simulink subsystem "simplePitch"  (R2024b)
settings: Solver=VariableStepAuto  StartTime=0.0  StopTime=10.0  RelTol=1e-3
settings Model: Creator=flyingtopher  LastModifiedBy=flyingtopher

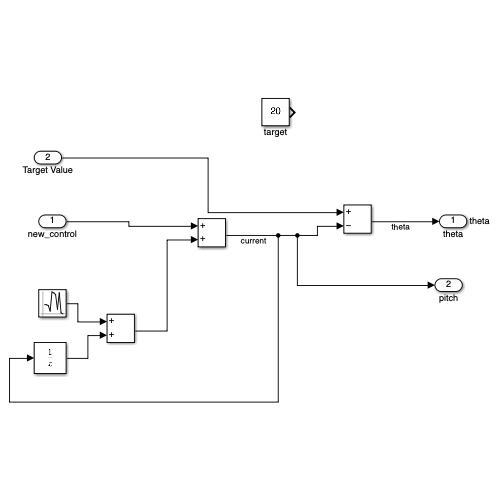
[thumbnail: Simulink's stored preview of the top-level diagram]
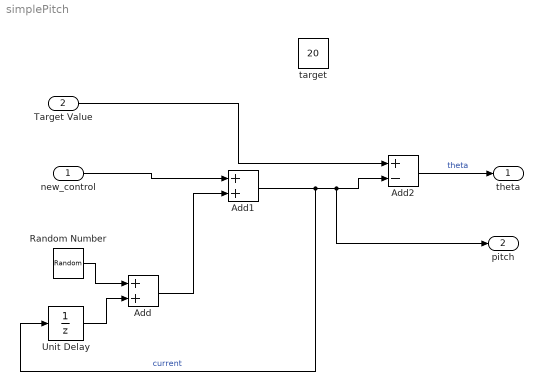
== system simplePitch ==
  new_control : Inport
  Target Value : Inport  Port=2
  Add : Sum
  Add1 : Sum
  Add2 : Sum  Inputs=+-
  Random Number : RandomNumber  Variance=0.5  SampleTime=0.1
  Unit Delay : UnitDelay  InitialCondition=3  SampleTime=-1  HasFrameUpgradeWarning=on
  target : Constant  Value=20
  theta : Outport  SignalName=theta
  pitch : Outport  Port=2
  wires:
  new_control/1 -> Add1/1
  Unit Delay/1 -> Add/2
  Random Number/1 -> Add/1
  Add/1 -> Add1/2
  Add1/1 -> Unit Delay/1, Add2/2, pitch/1  "current"
  Add2/1 -> theta/1  "theta"
  Target Value/1 -> Add2/1
